simulink model "rocky_motor_disturb_initial"  (R2022a)
settings: Solver=VariableStepAuto  StartTime=0.0  StopTime=2  RelTol=1e-3
model workspace (MAT data in the model file):
  m = 1000
values from neighbouring files (symbols this model uses):
  g = 9.81    [Rocky_closed_loop_poles.m]    (also in Rocky_closed_loop_poles_again.m; Rocky_closed_loop_poles_fresh_file.m; polederivation_CA.m; rocky_constants.m = 9.8)
  ki = 29095    [rocky_constants.m]
  kmotor = .63    (= 0.63)    [rocky_constants.m]
  kp = 5818.9    [rocky_constants.m]
  l = 0.4529    [Rocky_closed_loop_poles.m]    (also in Rocky_closed_loop_poles_again.m = 0.5588; Rocky_closed_loop_poles_fresh_file.m = 0.5588; polederivation_CA.m = 0.45; rocky_constants.m = 0.4)
  tau = .0325    (= 0.0325)    [rocky_constants.m]
settings Model: Creator=clee1  LastModifiedBy=ayydin
settings SolverCC: AlgebraicLoopSolver=TrustRegion
settings DebuggingCC: UnconnectedInputMsg=warning  UnconnectedOutputMsg=warning  UnconnectedLineMsg=warning  SFMachineParentedDataDiag=warning

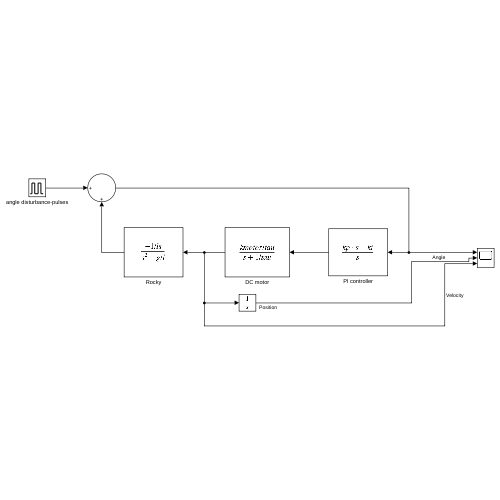
[thumbnail: Simulink's stored preview of the top-level diagram]
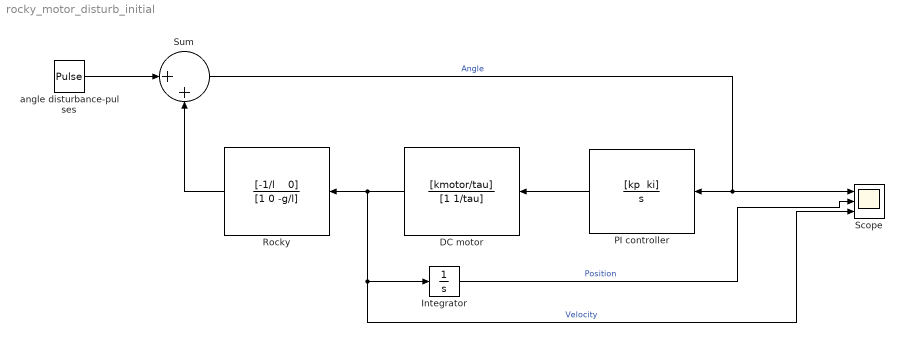
== system rocky_motor_disturb_initial ==
  DC motor : TransferFcn  Numerator=[kmotor/tau]  Denominator=[1 1/tau]
  Integrator : Integrator
  PI controller : TransferFcn  Numerator="[kp  ki]"  Denominator=[1 0 ]
  Rocky : TransferFcn  Numerator="[-1/l    0]"  Denominator=[1 0 -g/l]
  Scope : Scope  NumInputPorts=3
  Sum : Sum  Inputs=|++
  angle disturbance-pulses : DiscretePulseGenerator  PulseType=Time based  Amplitude=.1  Period=10  PulseWidth=.1  PhaseDelay=.5
  wires:
  Rocky/1 -> Sum/2
  Sum/1 -> Scope/1, PI controller/1  "Angle"
  angle disturbance-pulses/1 -> Sum/1
  DC motor/1 -> Integrator/1, Scope/3, Rocky/1  "Velocity"
  PI controller/1 -> DC motor/1
  Integrator/1 -> Scope/2  "Position"
